simulink model "ADK_longitudinal_controller"  (R2021a)
settings: configuration reference "ADK_IDS_Speedgoat" (kept outside this file)
undefined symbols (not defined in the file): CONTROL_CYCLE_TIME, DrivingMode, Gear, h, km, longitudinal_control_info, m, s, set_speed
libraries: simulink x3, pid_lib x1, aerolibconvert2 x1
settings Model: DataDictionary=ADK_IDS.sldd  Creator=xinrui  LastModifiedBy=Administrator
settings ConfigSetRef: SourceName=ADK_IDS_Speedgoat

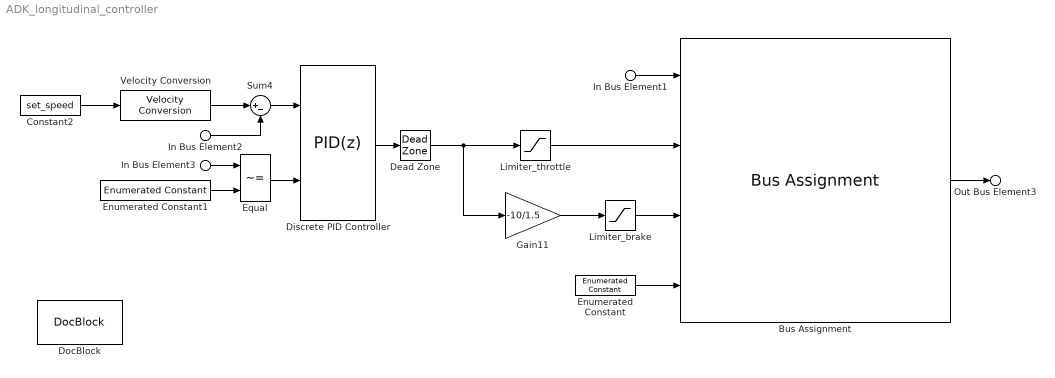
== system ADK_longitudinal_controller ==
  In Bus Element1 : Inport  PortName=InBus
  In Bus Element2 : Inport  PortName=InBus  Element=tram_info.speed.processed_value_current
  In Bus Element3 : Inport  PortName=InBus  Element=tram_info.driving_mode
  Bus Assignment : BusAssignment  AssignedSignals=longitudinal_control_info.set_throttle_pedal,longitudinal_control_info.set_brake_pedal,longitudinal_control_info.set_gear
  Constant2 : Constant  Value=set_speed  SampleTime=CONTROL_CYCLE_TIME
  Dead Zone : DeadZone  LowerValue=-10  UpperValue=1  SaturateOnIntegerOverflow=on
  Discrete PID Controller : pid_lib/PID Controller  Controller=PID  Form=Parallel  TimeDomain=Discrete-time  UseExternalTs=off  SampleTime=CONTROL_CYCLE_TIME  IntegratorMethod=Forward Euler  FilterMethod=Forward Euler  ControllerParametersSource=internal  P=20  I=0.3  D=3.065  UseFilter=off  N=100  TunerSelectOption=Transfer Function Based (PID Tuner App)  InitialConditionSource=internal  InitialConditionForIntegrator=0  InitialConditionForFilter=0  DifferentiatorICPrevScaledInput=0  ExternalReset=level  TrackingMode=off  Kt=1  LimitOutput=off  SatLimitsSource=internal  UpperSaturationLimit=inf  LowerSaturationLimit=-inf  LinearizeAsGain=off  AntiWindupMode=none  Kb=1  PGainOutDataTypeStr=double  PProdOutDataTypeStr=double  POutMin=[]  POutMax=[]  IGainOutDataTypeStr=double  IProdOutDataTypeStr=double  IOutMin=[-20]  IOutMax=[20]  DGainOutDataTypeStr=double  DProdOutDataTypeStr=double  DOutMin=[]  DOutMax=[]  NOutMin=[]  NOutMax=[]  SumOutDataTypeStr=double  SumOutMin=[]  SumOutMax=[]  SaturationOutMin=[]  SaturationOutMax=[]  PParamMin=[]  PParamMax=[]  IParamMin=[]  IParamMax=[]  DParamMin=[]  DParamMax=[]  NParamMin=[]  NParamMax=[]  KbParamMin=[]  KbParamMax=[]  KtParamMin=[]  KtParamMax=[]  KbOutMin=[]  KbOutMax=[]  KtOutMin=[]  KtOutMax=[]  IntegratorOutMin=[]  IntegratorOutMax=[]  FilterOutMin=[]  FilterOutMax=[]  SumI1OutMin=[]  SumI1OutMax=[]  SumI2OutMin=[]  SumI2OutMax=[]  SumI3OutMin=[]  SumI3OutMax=[]  SumI4OutMin=[]  SumI4OutMax=[]  SumDOutMin=[]  SumDOutMax=[]  DifferentiatorOutMin=[]  DifferentiatorOutMax=[]  FilterDiffOutCoefMin=[]  FilterDiffOutCoefMax=[]  ReciprocalOutMin=[]  ReciprocalOutMax=[]  SumDenOutMin=[]  SumDenOutMax=[]  SumNumOutMin=[]  SumNumOutMax=[]  DivideOutMin=[]  DivideOutMax=[]  UdiffTsProdOutMin=[]  UdiffTsProdOutMax=[]  NTsProdOutMin=[]  NTsProdOutMax=[]  UintegralTsProdOutMin=[]  UintegralTsProdOutMax=[]  UngainTsProdOutMin=[]  UngainTsProdOutMax=[]  IntegratorContinuousStateAttributes=''  IntegratorStateMustResolveToSignalObject=off  IntegratorRTWStateStorageClass=Auto  FilterContinuousStateAttributes=''  FilterStateMustResolveToSignalObject=off  FilterRTWStateStorageClass=Auto  ParallelPVariant=InternalParameters  IdealPVariant=Disabled  IVariant=InternalParameters  DVariant=InternalParameters  IntegratorVariant=Discrete  SatVariant=Disabled  AWVariant=Passthrough  PCopyVariant=Disabled  TRVariant=Disabled  FdbkBlocksVariant=Forward  IdealPFdbkVariant=Disabled  SatFdbkVariant=Disabled  DerivativeFilterVariant=Differentiator  NVariant=Passthrough  NCopyVariant=Disabled_SignalSpec  FilterICVariant=InternalICsDifferentiator  IntegratorICVariant=InternalICs  ExternalResetVariant=ExternalReset  TRSumVariant=Passthrough  SumFdbkVariant=Disabled  SumVariant=Sum_PID  TsampFilterVariant=InternalTs  TsampNgainVariant=Passthrough  TsampIntegralVariant=Passthrough  ExternalSaturationOutDataTypeStr=Inherit: Same as second input
  DocBlock : simulink/Model-Wide Utilities/DocBlock  DocumentType=HTML  mask(DocBlock){}
      mask Display:
      | plot([.8 0 0 1 1 .8 .8 1],[1 1 0 0 .8 1 .8 .8]);
      | text(.5,.6,'CHANGELOG','horizontalalignment','center');
      | text(.95,.05,get_param(gcb,'DocumentType'),'verticalalignment','bottom','horizontalalignment','right');
  Enumerated Constant : simulink/Sources/Enumerated Constant  OutDataTypeStr=Enum: Gear  Value=Gear.D  SampleTime=CONTROL_CYCLE_TIME
  Enumerated Constant1 : simulink/Sources/Enumerated Constant  OutDataTypeStr=Enum: DrivingMode  Value=DrivingMode.Autopilot  SampleTime=CONTROL_CYCLE_TIME
  Equal : RelationalOperator  Operator=~=  OutDataTypeStr=boolean  RndMeth=Simplest
  Gain11 : Gain  Gain=-10/1.5
  Limiter_brake : Saturate  UpperLimit=100  LowerLimit=0
  Limiter_throttle : Saturate  UpperLimit=100  LowerLimit=0
  Sum4 : Sum  Inputs=|+-
  Velocity Conversion : aerolibconvert2/Velocity Conversion  IU=km/h  OU=m/s
  Out Bus Element3 : Outport  PortName=OutBus
  wires:
  In Bus Element2/1 -> Sum4/2
  Enumerated Constant/1 -> Bus Assignment/4
  Bus Assignment/1 -> Out Bus Element3/1
  In Bus Element1/1 -> Bus Assignment/1
  Velocity Conversion/1 -> Sum4/1
  Dead Zone/1 -> Limiter_throttle/1, Gain11/1
  Limiter_throttle/1 -> Bus Assignment/2
  Limiter_brake/1 -> Bus Assignment/3
  Gain11/1 -> Limiter_brake/1
  Discrete PID Controller/1 -> Dead Zone/1
  Sum4/1 -> Discrete PID Controller/1
  Enumerated Constant1/1 -> Equal/2
  In Bus Element3/1 -> Equal/1
  Equal/1 -> Discrete PID Controller/2
  Constant2/1 -> Velocity Conversion/1
